simulink subsystem "Controller"  (R2022b)
settings: Solver=VariableStepAuto  StartTime=0.0  StopTime=10.0  RelTol=1e-3
undefined symbols (not defined in the file or in its folder): control, DiscIntNeverNeededParam, magnetorquers, sat, sensors, settings
libraries: simulink x3, matrix_library x3, vrlib x3, cstblocks x2
settings Model: Creator=brent  LastModifiedBy=brent

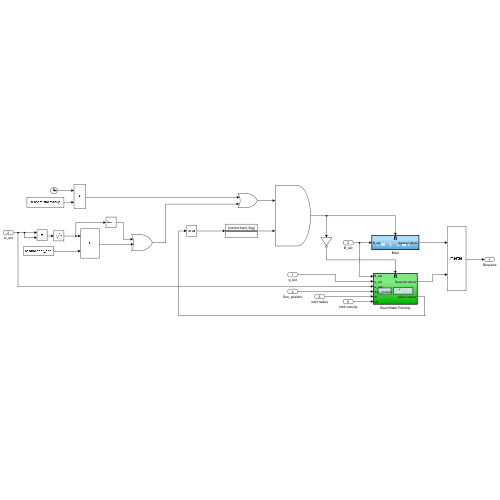
[thumbnail: Simulink's stored preview of the top-level diagram]
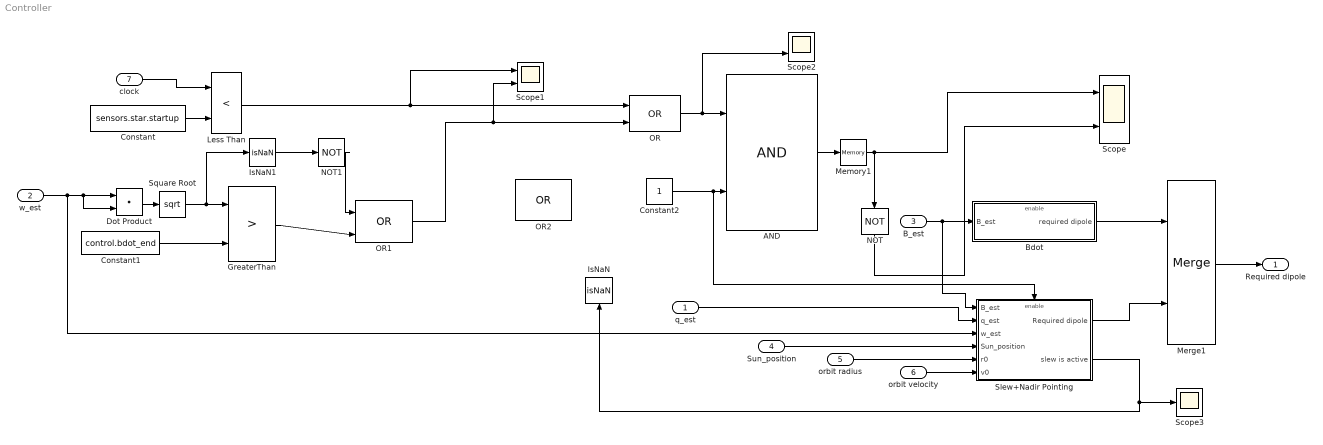
== system Controller ==
  q_est : Inport
  w_est : Inport  Port=2
  B_est : Inport  Port=3
  Sun_position : Inport  Port=4
  orbit radius : Inport  Port=5
  orbit velocity : Inport  Port=6
  clock : Inport  Port=7
  AND : Logic  IconShape=distinctive  AllPortsSameDT=off  OutDataTypeStr=boolean
  Bdot : Subsystem  TreatAsAtomicUnit=on
  Constant : Constant  Value=sensors.star.startup
  Constant1 : Constant  Value=control.bdot_end
  Constant2 : Constant
  Dot Product : DotProduct  OutDataTypeStr=Inherit: Inherit via internal rule
  GreaterThan : RelationalOperator  Operator=>  OutDataTypeStr=boolean  RndMeth=Simplest  InputSameDT=off
  IsNaN : RelationalOperator  Operator=isNaN  OutDataTypeStr=boolean  RndMeth=Simplest  InputSameDT=off
  IsNaN1 : RelationalOperator  Operator=isNaN  OutDataTypeStr=boolean  RndMeth=Simplest  InputSameDT=off
  Less Than : RelationalOperator  Operator=<  OutDataTypeStr=boolean  RndMeth=Simplest  InputSameDT=off
  Memory1 : Memory  InitialCondition=true  InheritSampleTime=on
  Merge1 : Merge
  NOT : Logic  Operator=NOT  IconShape=distinctive  AllPortsSameDT=off  OutDataTypeStr=boolean
  NOT1 : Logic  Operator=NOT  IconShape=distinctive  AllPortsSameDT=off  OutDataTypeStr=boolean
  OR : Logic  Operator=OR  IconShape=distinctive  AllPortsSameDT=off  OutDataTypeStr=boolean
  OR1 : Logic  Operator=OR  IconShape=distinctive  AllPortsSameDT=off  OutDataTypeStr=boolean
  OR2 : Logic  Operator=OR  IconShape=distinctive  AllPortsSameDT=off  OutDataTypeStr=boolean
  Scope : Scope  NumInputPorts=2
  Scope1 : Scope  NumInputPorts=2
  Scope2 : Scope  NumInputPorts=2
  Scope3 : Scope
  Slew+Nadir Pointing : Subsystem
  Square Root : Sqrt
  Required dipole : Outport
  wires:
  q_est/1 -> Slew+Nadir Pointing/2(q_est)
  w_est/1 -> Slew+Nadir Pointing/3(w_est), Dot Product/2, Dot Product/1
  Constant/1 -> Less Than/2
  Less Than/1 -> OR/1, Scope1/1
  Dot Product/1 -> Square Root/1
  Square Root/1 -> GreaterThan/1, IsNaN1/1
  Constant1/1 -> GreaterThan/2
  Slew+Nadir Pointing/2(slew is active) -> IsNaN/1, Scope3/1
  OR/1 -> AND/1, Scope2/2
  GreaterThan/1 -> OR1/2
  OR1/1 -> OR/2, Scope1/2
  Slew+Nadir Pointing/1(Required dipole) -> Merge1/2
  Merge1/1 -> Required dipole/1
  B_est/1 -> Slew+Nadir Pointing/1(B_est), Bdot/1(B_est)
  Bdot/1(required dipole) -> Merge1/1
  NOT/1 -> Scope/2
  Sun_position/1 -> Slew+Nadir Pointing/4(Sun_position)
  orbit radius/1 -> Slew+Nadir Pointing/5(r0)
  orbit velocity/1 -> Slew+Nadir Pointing/6(v0)
  clock/1 -> Less Than/1
  AND/1 -> Memory1/1
  Memory1/1 -> Scope/1, NOT/1
  Constant2/1 -> AND/2, Slew+Nadir Pointing/Enable
  IsNaN1/1 -> NOT1/1
  NOT1/1 -> OR1/1

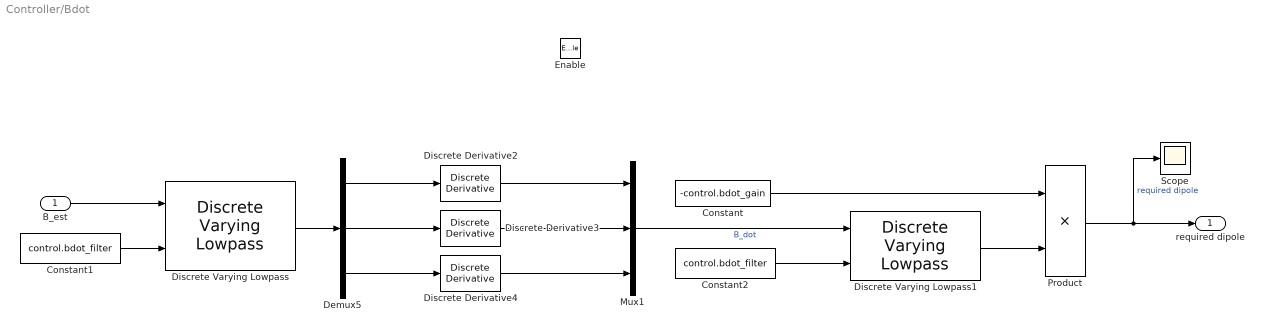
== system Controller/Bdot ==
  B_est : Inport
  Enable : EnablePort
  Constant : Constant  Value=-control.bdot_gain
  Constant1 : Constant  Value=control.bdot_filter  SampleTime=-1
  Constant2 : Constant  Value=control.bdot_filter  SampleTime=-1
  Demux5 : Demux  Outputs=3
  Discrete Derivative2 : simulink/Discrete/Discrete Derivative  gainval=1.0  ICPrevScaledInput=0  OutMin=[]  OutMax=[]  OutDataType=fixdt(1, 16)  OutScaling=2^-10  DoSatur=off
  Discrete Derivative3 : simulink/Discrete/Discrete Derivative  gainval=1.0  ICPrevScaledInput=0  OutMin=[]  OutMax=[]  OutDataType=fixdt(1, 16)  OutScaling=2^-10  DoSatur=off
  Discrete Derivative4 : simulink/Discrete/Discrete Derivative  gainval=1.0  ICPrevScaledInput=0  OutMin=[]  OutMax=[]  OutDataType=fixdt(1, 16)  OutScaling=2^-10  DoSatur=off
  Discrete Varying Lowpass : cstblocks/Linear Parameter Varying/Discrete Varying Lowpass  N=1  w0=0  Ts=1/sensors.star.frequency
  Discrete Varying Lowpass1 : cstblocks/Linear Parameter Varying/Discrete Varying Lowpass  N=1  w0=0  Ts=1/sensors.star.frequency
  Mux1 : Mux  Inputs=3
  Product : Product
  Scope : Scope
  required dipole : Outport
  wires:
  Discrete Derivative2/1 -> Mux1/1
  Demux5/2 -> Discrete Derivative3/1
  Constant1/1 -> Discrete Varying Lowpass/2
  Demux5/1 -> Discrete Derivative2/1
  Demux5/3 -> Discrete Derivative4/1
  Discrete Derivative3/1 -> Mux1/2
  Discrete Derivative4/1 -> Mux1/3
  Discrete Varying Lowpass1/1 -> Product/2
  Product/1 -> required dipole/1, Scope/1  "required dipole"
  Constant/1 -> Product/1
  Discrete Varying Lowpass/1 -> Demux5/1
  B_est/1 -> Discrete Varying Lowpass/1
  Constant2/1 -> Discrete Varying Lowpass1/2
  Mux1/1 -> Discrete Varying Lowpass1/1  "B_dot"

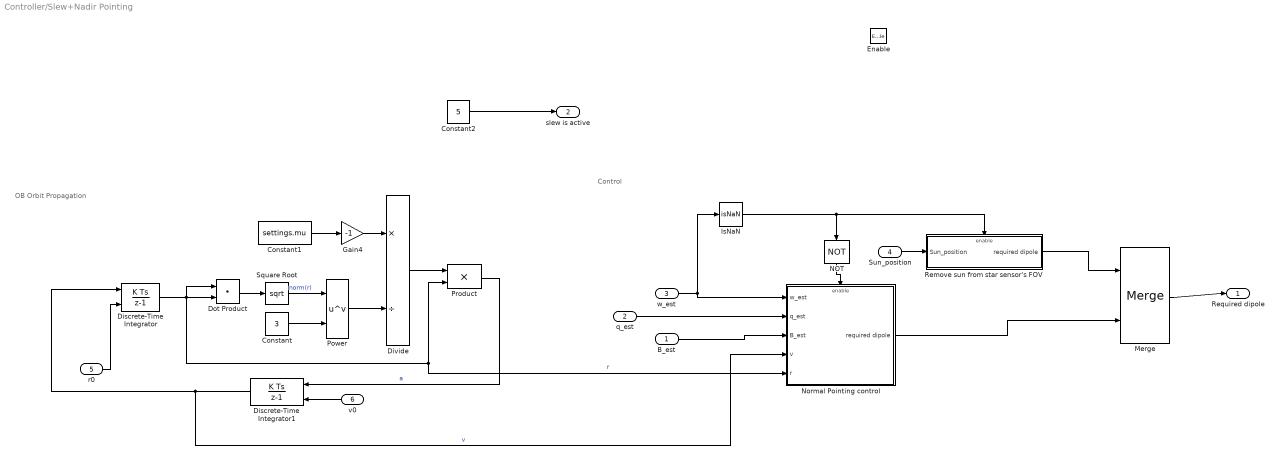
== system Controller/Slew+Nadir Pointing ==
  note: Control
  note: OB Orbit Propagation
  B_est : Inport
  q_est : Inport  Port=2
  w_est : Inport  Port=3
  Sun_position : Inport  Port=4
  r0 : Inport  Port=5
  v0 : Inport  Port=6
  Enable : EnablePort
  Constant : Constant  Value=3
  Constant1 : Constant  Value=settings.mu
  Constant2 : Constant  Value=5
  Discrete-Time Integrator : DiscreteIntegrator  InitialConditionSource=external  InitialCondition=settings.r0  SampleTime=-1  ICPrevOutput=DiscIntNeverNeededParam  ICPrevScaledInput=DiscIntNeverNeededParam
  Discrete-Time Integrator1 : DiscreteIntegrator  InitialConditionSource=external  InitialCondition=settings.v0  SampleTime=-1  ICPrevOutput=DiscIntNeverNeededParam  ICPrevScaledInput=DiscIntNeverNeededParam
  Divide : Product  Inputs=*/
  Dot Product : DotProduct  OutDataTypeStr=Inherit: Inherit via internal rule
  Gain4 : Gain  Gain=-1
  IsNaN : RelationalOperator  Operator=isNaN  OutDataTypeStr=boolean  RndMeth=Simplest  InputSameDT=off
  Merge : Merge
  NOT : Logic  Operator=NOT  IconShape=distinctive  AllPortsSameDT=off  OutDataTypeStr=boolean
  Normal Pointing control : Subsystem
  Power : Math  Operator=pow
  Product : Product
  Remove sun from star sensor's FOV : Subsystem  TreatAsAtomicUnit=on
  Square Root : Sqrt
  Required dipole : Outport
  slew is active : Outport  Port=2
  wires:
  Constant2/1 -> slew is active/1
  Gain4/1 -> Divide/1
  Discrete-Time Integrator/1 -> Product/2, Normal Pointing control/5(r), Dot Product/2, Dot Product/1  "r"
  Constant1/1 -> Gain4/1
  Power/1 -> Divide/2
  Discrete-Time Integrator1/1 -> Discrete-Time Integrator/1, Normal Pointing control/4(v)  "v"
  Dot Product/1 -> Square Root/1
  Constant/1 -> Power/2
  Square Root/1 -> Power/1  "norm(r)"
  Divide/1 -> Product/1
  Product/1 -> Discrete-Time Integrator1/1  "a"
  q_est/1 -> Normal Pointing control/2(q_est)
  w_est/1 -> IsNaN/1, Normal Pointing control/1(w_est)
  NOT/1 -> Normal Pointing control/Enable
  IsNaN/1 -> Remove sun from star sensor's FOV/Enable, NOT/1
  Sun_position/1 -> Remove sun from star sensor's FOV/1(Sun_position)
  Remove sun from star sensor's FOV/1(required dipole) -> Merge/1
  Normal Pointing control/1(required dipole) -> Merge/2
  B_est/1 -> Normal Pointing control/3(B_est)
  Merge/1 -> Required dipole/1
  r0/1 -> Discrete-Time Integrator/2
  v0/1 -> Discrete-Time Integrator1/2

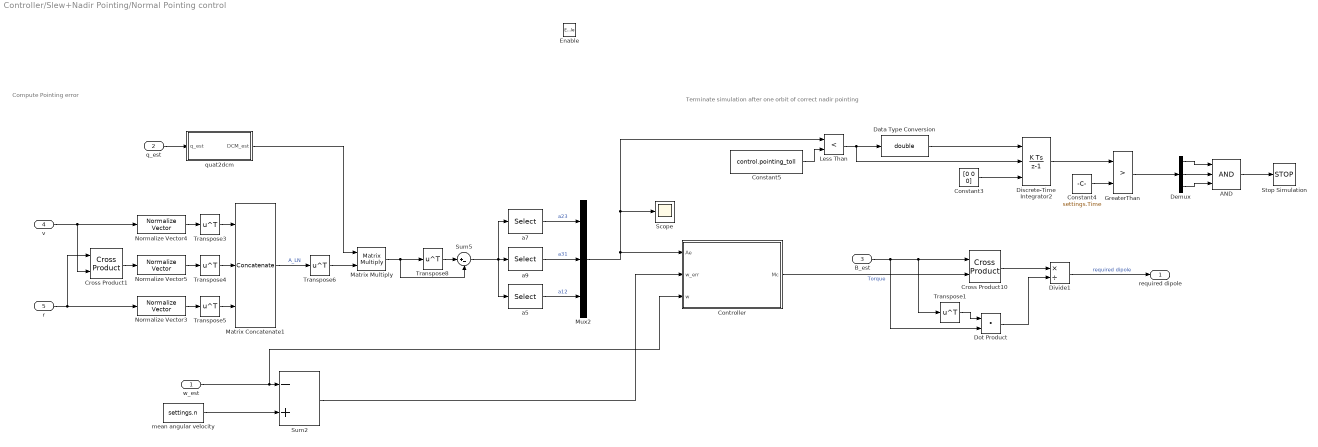
== system Controller/Slew+Nadir Pointing/Normal Pointing control ==
  note: Terminate simulation after one orbit of correct nadir pointing
  note: Compute Pointing error
  w_est : Inport
  q_est : Inport  Port=2
  B_est : Inport  Port=3
  v : Inport  Port=4
  r : Inport  Port=5
  Enable : EnablePort
  AND : Logic  Inputs=3  IconShape=distinctive  AllPortsSameDT=off  OutDataTypeStr=boolean
  Constant3 : Constant  Value=[0 0 0]
  Constant4 : Constant  Value=settings.Time
  Constant5 : Constant  Value=control.pointing_toll
  "Controller " : Subsystem  TreatAsAtomicUnit=on  SystemSampleTime=1
  Cross Product1 : matrix_library/Cross Product
  Cross Product10 : matrix_library/Cross Product
  Data Type Conversion : DataTypeConversion  OutDataTypeStr=double  SaturateOnIntegerOverflow=off  RndMeth=Floor
  Demux : Demux  Outputs=3
  Discrete-Time Integrator2 : DiscreteIntegrator  ExternalReset=either  InitialConditionSource=external  ICPrevOutput=DiscIntNeverNeededParam  ICPrevScaledInput=DiscIntNeverNeededParam
  Divide1 : Product  Inputs=*/  RndMeth=Zero  SaturateOnIntegerOverflow=on
  Dot Product : DotProduct  OutDataTypeStr=Inherit: Inherit via internal rule
  GreaterThan : RelationalOperator  Operator=>  OutDataTypeStr=boolean  RndMeth=Simplest  InputSameDT=off
  Less Than : RelationalOperator  Operator=<  OutDataTypeStr=boolean  RndMeth=Simplest  InputSameDT=off
  Matrix Concatenate1 : Concatenate  NumInputs=3  Mode=Multidimensional array
  Matrix Multiply : Product  Multiplication=Matrix(*)
  Mux2 : Mux  Inputs=3
  Normalize Vector3 : vrlib/Utilities/Normalize Vector  maxzero=0
  Normalize Vector4 : vrlib/Utilities/Normalize Vector  maxzero=0
  Normalize Vector5 : vrlib/Utilities/Normalize Vector  maxzero=0
  Scope : Scope
  Stop Simulation : Stop
  Sum2 : Sum  Inputs=-+
  Sum5 : Sum  Inputs=|+-
  Transpose{1,3..6,8} (6 alike) : Math  Operator=transpose
  a5 : Selector  NumberOfDimensions=2  InputPortWidth=3  IndexOptions=Index vector (dialog),Index vector (dialog)  Indices=1,2  OutputSizes=1,1
  a7 : Selector  NumberOfDimensions=2  InputPortWidth=3  IndexOptions=Index vector (dialog),Index vector (dialog)  Indices=2,3  OutputSizes=1,1
  a9 : Selector  NumberOfDimensions=2  InputPortWidth=3  IndexOptions=Index vector (dialog),Index vector (dialog)  Indices=3,1  OutputSizes=1,1
  mean angular velocity : Constant  Value=settings.n
  quat2dcm : Subsystem
  required dipole : Outport
  wires:
  Transpose8/1 -> Sum5/1
  Constant5/1 -> Less Than/2
  Transpose4/1 -> Matrix Concatenate1/2
  v/1 -> Normalize Vector4/1, Cross Product1/2
  Sum5/1 -> a7/1, a9/1, a5/1
  Matrix Multiply/1 -> Transpose8/1, Sum5/2
  Cross Product1/1 -> Normalize Vector5/1
  Normalize Vector5/1 -> Transpose4/1
  Constant4/1 -> GreaterThan/2
  Transpose5/1 -> Matrix Concatenate1/3
  a9/1 -> Mux2/2  "a31"
  Normalize Vector4/1 -> Transpose3/1
  AND/1 -> Stop Simulation/1
  quat2dcm/1(DCM_est) -> Matrix Multiply/1
  Transpose3/1 -> Matrix Concatenate1/1
  a5/1 -> Mux2/3  "a12"
  r/1 -> Cross Product1/1, Normalize Vector3/1
  a7/1 -> Mux2/1  "a23"
  Discrete-Time Integrator2/1 -> GreaterThan/1
  Sum2/1 -> "Controller "/2(w_err)
  Transpose6/1 -> Matrix Multiply/2
  Mux2/1 -> "Controller "/1(Ae), Less Than/1, Scope/1
  w_est/1 -> Sum2/1, "Controller "/3(w)
  mean angular velocity/1 -> Sum2/2
  Less Than/1 -> Discrete-Time Integrator2/2, Data Type Conversion/1
  Demux/1 -> AND/1
  Data Type Conversion/1 -> Discrete-Time Integrator2/1
  Normalize Vector3/1 -> Transpose5/1
  Demux/2 -> AND/2
  Matrix Concatenate1/1 -> Transpose6/1  "A_LN"
  q_est/1 -> quat2dcm/1(q_est)
  Demux/3 -> AND/3
  GreaterThan/1 -> Demux/1
  Constant3/1 -> Discrete-Time Integrator2/3
  "Controller "/1(Mc) -> Cross Product10/2  "Torque"
  Dot Product/1 -> Divide1/2
  Cross Product10/1 -> Divide1/1
  Divide1/1 -> required dipole/1  "required dipole"
  B_est/1 -> Dot Product/2, Cross Product10/1, Transpose1/1
  Transpose1/1 -> Dot Product/1

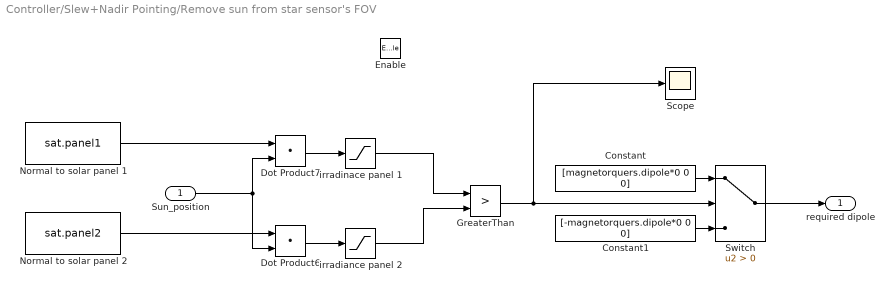
== system Controller/Slew+Nadir Pointing/Remove sun from star sensor's FOV ==
  Sun_position : Inport
  Enable : EnablePort
  Constant : Constant  Value=[magnetorquers.dipole*0 0 0]
  Constant1 : Constant  Value=[-magnetorquers.dipole*0 0 0]
  Dot Product6 : DotProduct  OutDataTypeStr=Inherit: Inherit via internal rule
  Dot Product7 : DotProduct  OutDataTypeStr=Inherit: Inherit via internal rule
  GreaterThan : RelationalOperator  Operator=>  OutDataTypeStr=boolean  RndMeth=Simplest  InputSameDT=off
  Normal to solar panel 1 : Constant  Value=sat.panel1
  Normal to solar panel 2 : Constant  Value=sat.panel2
  Scope : Scope
  Switch : Switch  Criteria=u2 > Threshold  SaturateOnIntegerOverflow=off  InputSameDT=off
  irradiance panel 2 : Saturate  UpperLimit=1  LowerLimit=0
  irradinace panel 1 : Saturate  UpperLimit=1  LowerLimit=0
  required dipole : Outport
  wires:
  Sun_position/1 -> Dot Product7/2, Dot Product6/2
  Dot Product6/1 -> irradiance panel 2/1
  Dot Product7/1 -> irradinace panel 1/1
  irradinace panel 1/1 -> GreaterThan/1
  Normal to solar panel 2/1 -> Dot Product6/1
  Normal to solar panel 1/1 -> Dot Product7/1
  irradiance panel 2/1 -> GreaterThan/2
  GreaterThan/1 -> Switch/2, Scope/1
  Switch/1 -> required dipole/1
  Constant/1 -> Switch/1
  Constant1/1 -> Switch/3

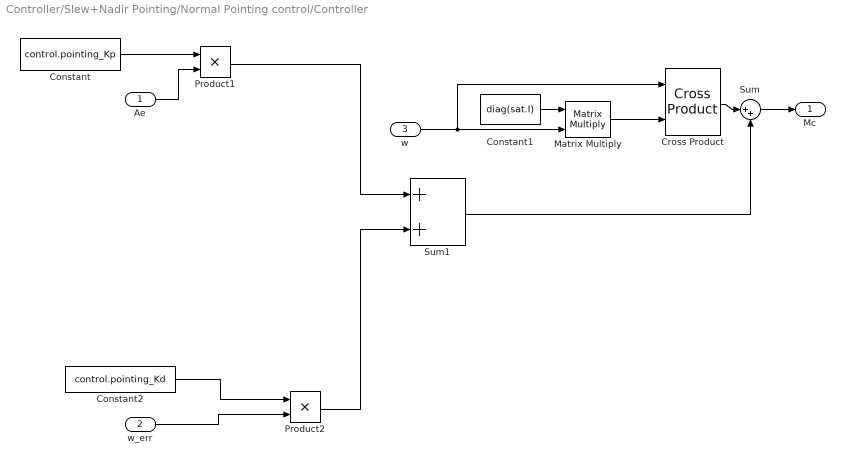
== system Controller/Slew+Nadir Pointing/Normal Pointing control/Controller  ==
  Ae : Inport
  w_err : Inport  Port=2
  w : Inport  Port=3
  Constant : Constant  Value=control.pointing_Kp
  Constant1 : Constant  Value=diag(sat.I)
  Constant2 : Constant  Value=control.pointing_Kd
  Cross Product : matrix_library/Cross Product
  Matrix Multiply : Product  Multiplication=Matrix(*)
  Product1 : Product
  Product2 : Product
  Sum : Sum  Inputs=|++
  Sum1 : Sum
  Mc : Outport
  wires:
  Sum1/1 -> Sum/2
  w/1 -> Cross Product/1, Matrix Multiply/2
  Constant1/1 -> Matrix Multiply/1
  Matrix Multiply/1 -> Cross Product/2
  Cross Product/1 -> Sum/1
  Sum/1 -> Mc/1
  w_err/1 -> Product2/2
  Ae/1 -> Product1/2
  Constant/1 -> Product1/1
  Product2/1 -> Sum1/2
  Constant2/1 -> Product2/1
  Product1/1 -> Sum1/1

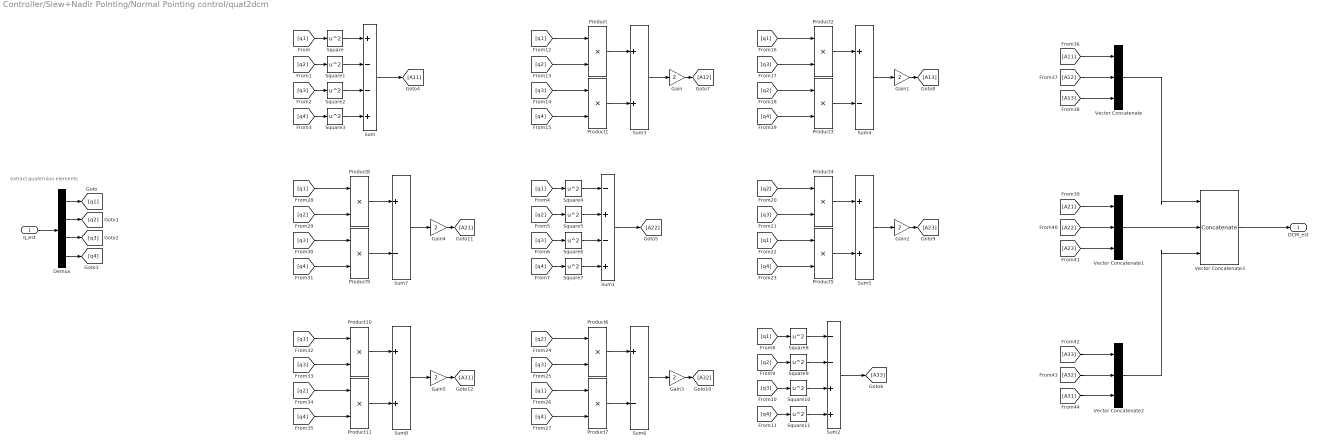
== system Controller/Slew+Nadir Pointing/Normal Pointing control/quat2dcm ==
  note: extract quaternion elements
  q_est : Inport
  Demux : Demux
  Gain{,1..5} (6 alike) : Gain  Gain=2
  Product{,1..11} (12 alike) : Product
  Square{,1..11} (12 alike) : Math  Operator=square
  Sum : Sum  Inputs=+--+
  Sum1 : Sum  Inputs=-+-+
  Sum2 : Sum  Inputs=--++
  Sum3 : Sum
  Sum4 : Sum  Inputs=+-
  Sum5 : Sum
  Sum6 : Sum  Inputs=+-
  Sum7 : Sum  Inputs=+-
  Sum8 : Sum
  Vector Concatenate : Concatenate  NumInputs=3  Mode=Multidimensional array  ConcatenateDimension=2
  Vector Concatenate1 : Concatenate  NumInputs=3  Mode=Multidimensional array  ConcatenateDimension=2
  Vector Concatenate2 : Concatenate  NumInputs=3  Mode=Multidimensional array  ConcatenateDimension=2
  Vector Concatenate3 : Concatenate  NumInputs=3  Mode=Multidimensional array
  DCM_est : Outport
  wires:
  q_est/1 -> Demux/1
  Demux/1 -> [q1]
  Demux/2 -> [q2]
  Demux/3 -> [q3]
  Demux/4 -> [q4]
  [q1] -> Square/1
  [q2] -> Square1/1
  [q3] -> Square2/1
  [q4] -> Square3/1
  Square3/1 -> Sum/4
  Square2/1 -> Sum/3
  Square1/1 -> Sum/2
  Square/1 -> Sum/1
  Sum/1 -> [A11]
  Sum1/1 -> [A22]
  Square4/1 -> Sum1/1
  Square5/1 -> Sum1/2
  Square6/1 -> Sum1/3
  Square7/1 -> Sum1/4
  [q4] -> Square7/1
  [q3] -> Square6/1
  [q2] -> Square5/1
  [q1] -> Square4/1
  [q1] -> Square8/1
  [q2] -> Square9/1
  [q3] -> Square10/1
  [q4] -> Square11/1
  Square11/1 -> Sum2/4
  Square10/1 -> Sum2/3
  Square9/1 -> Sum2/2
  Square8/1 -> Sum2/1
  Sum2/1 -> [A33]
  [q1] -> Product/1
  [q2] -> Product/2
  [q3] -> Product1/1
  [q4] -> Product1/2
  Product1/1 -> Sum3/2
  Product/1 -> Sum3/1
  Sum3/1 -> Gain/1
  Gain/1 -> [A12]
  Gain1/1 -> [A13]
  Sum4/1 -> Gain1/1
  Product2/1 -> Sum4/1
  Product3/1 -> Sum4/2
  [q4] -> Product3/2
  [q2] -> Product3/1
  [q3] -> Product2/2
  [q1] -> Product2/1
  [q2] -> Product4/1
  [q3] -> Product4/2
  [q1] -> Product5/1
  [q4] -> Product5/2
  Product5/1 -> Sum5/2
  Product4/1 -> Sum5/1
  Sum5/1 -> Gain2/1
  Gain2/1 -> [A23]
  Gain3/1 -> [A32]
  Sum6/1 -> Gain3/1
  Product6/1 -> Sum6/1
  Product7/1 -> Sum6/2
  [q4] -> Product7/2
  [q1] -> Product7/1
  [q3] -> Product6/2
  [q2] -> Product6/1
  Gain4/1 -> [A21]
  Sum7/1 -> Gain4/1
  Product8/1 -> Sum7/1
  Product9/1 -> Sum7/2
  [q4] -> Product9/2
  [q3] -> Product9/1
  [q2] -> Product8/2
  [q1] -> Product8/1
  [q1] -> Product10/1
  [q3] -> Product10/2
  [q2] -> Product11/1
  [q4] -> Product11/2
  Product11/1 -> Sum8/2
  Product10/1 -> Sum8/1
  Sum8/1 -> Gain5/1
  Gain5/1 -> [A31]
  [A12] -> Vector Concatenate/2
  [A13] -> Vector Concatenate/3
  [A11] -> Vector Concatenate/1
  [A21] -> Vector Concatenate1/1
  [A22] -> Vector Concatenate1/2
  [A23] -> Vector Concatenate1/3
  [A33] -> Vector Concatenate2/1
  [A32] -> Vector Concatenate2/2
  [A31] -> Vector Concatenate2/3
  Vector Concatenate1/1 -> Vector Concatenate3/2
  Vector Concatenate2/1 -> Vector Concatenate3/3
  Vector Concatenate/1 -> Vector Concatenate3/1
  Vector Concatenate3/1 -> DCM_est/1
